simulink model "Reflex_Ursino"  (Simulink 6.4)
settings: Solver=ode45  StartTime=0.0  StopTime=10.0  RelTol=1e-3
values from neighbouring files (symbols this model uses):
  fapIC = 4.4492    [Reflex_Ursino_IC.m]    (also in Respiratory_IC.m)
  fcs_max = 47.78    [Cardiovascular_IC.m]    (also in Reflex_Ursino_IC.m)
  fcs_min = 2.52    [Cardiovascular_IC.m]    (also in Reflex_Ursino_IC.m)
  k_cs = 11.758    [Cardiovascular_IC.m]    (also in Reflex_Ursino_IC.m)
  Pn = 90    [Cardiovascular_IC.m]    (also in Reflex_Ursino_IC.m)
settings Model: LastModifiedBy=CLM
settings OptimizationCC: BlockReduction=off  BooleanDataType=off
settings DebuggingCC: SolverPrmCheckMsg=none  StrictBusMsg=None
settings HardwareCC: TargetUnknown=on

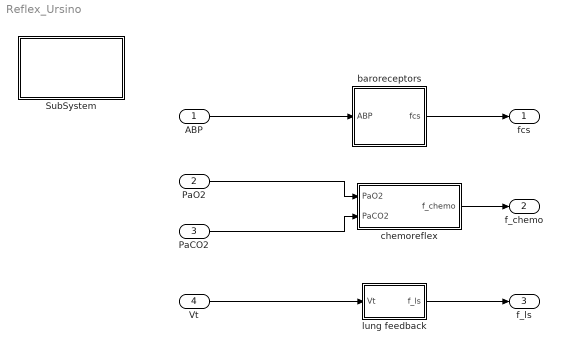
== system Reflex_Ursino ==
  ABP : Inport
  PaO2 : Inport  Port=2
  PaCO2 : Inport  Port=3
  Vt : Inport  Port=4
  SubSystem : Subsystem
      settings: OpenFcn=Reflex_Ursino_IC
      mask Display: disp('"double click here"\n to load \nReflex_Ursino \ninitial values');
  baroreceptors : Subsystem
  chemoreflex : Subsystem
  lung feedback : Subsystem
  fcs : Outport
  f_chemo : Outport  Port=2
  f_ls : Outport  Port=3
  wires:
  baroreceptors/1(fcs) -> fcs/1
  ABP/1 -> baroreceptors/1(ABP)
  chemoreflex/1(f_chemo) -> f_chemo/1
  PaCO2/1 -> chemoreflex/2(PaCO2)
  PaO2/1 -> chemoreflex/1(PaO2)
  Vt/1 -> lung feedback/1(Vt)
  lung feedback/1(f_ls) -> f_ls/1

== system Reflex_Ursino/SubSystem ==

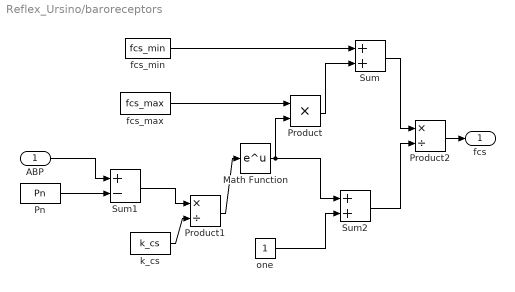
== system Reflex_Ursino/baroreceptors ==
  ABP : Inport
  Math Function : Math  SaturateOnIntegerOverflow=on
  Pn : Constant  Value=Pn  OutDataType=sfix(16)  ConRadixGroup=Use specified scaling  OutScaling=2^0  SampleTime=inf  FramePeriod=inf
  Product : Product  SaturateOnIntegerOverflow=on  RndMeth=Zero  InputSameDT=on
  Product1 : Product  Inputs=*/  SaturateOnIntegerOverflow=on  RndMeth=Zero  InputSameDT=on
  Product2 : Product  Inputs=*/  SaturateOnIntegerOverflow=on  RndMeth=Zero  InputSameDT=on
  Sum : Sum  SaturateOnIntegerOverflow=on  InputSameDT=on
  Sum1 : Sum  Inputs=+-  SaturateOnIntegerOverflow=on  InputSameDT=on
  Sum2 : Sum  SaturateOnIntegerOverflow=on  InputSameDT=on
  fcs_max : Constant  Value=fcs_max  OutDataType=sfix(16)  ConRadixGroup=Use specified scaling  OutScaling=2^0  SampleTime=inf  FramePeriod=inf
  fcs_min : Constant  Value=fcs_min  OutDataType=sfix(16)  ConRadixGroup=Use specified scaling  OutScaling=2^0  SampleTime=inf  FramePeriod=inf
  k_cs : Constant  Value=k_cs  OutDataType=sfix(16)  ConRadixGroup=Use specified scaling  OutScaling=2^0  SampleTime=inf  FramePeriod=inf
  one : Constant  Value=1  OutDataType=sfix(16)  ConRadixGroup=Use specified scaling  OutScaling=2^0  SampleTime=inf  FramePeriod=inf
  fcs : Outport
  wires:
  Sum1/1 -> Product1/1
  Product2/1 -> fcs/1
  Product/1 -> Sum/2
  Sum2/1 -> Product2/2
  Sum/1 -> Product2/1
  one/1 -> Sum2/2
  Math Function/1 -> Sum2/1, Product/2
  Product1/1 -> Math Function/1
  k_cs/1 -> Product1/2
  fcs_max/1 -> Product/1
  fcs_min/1 -> Sum/1
  Pn/1 -> Sum1/2
  ABP/1 -> Sum1/1

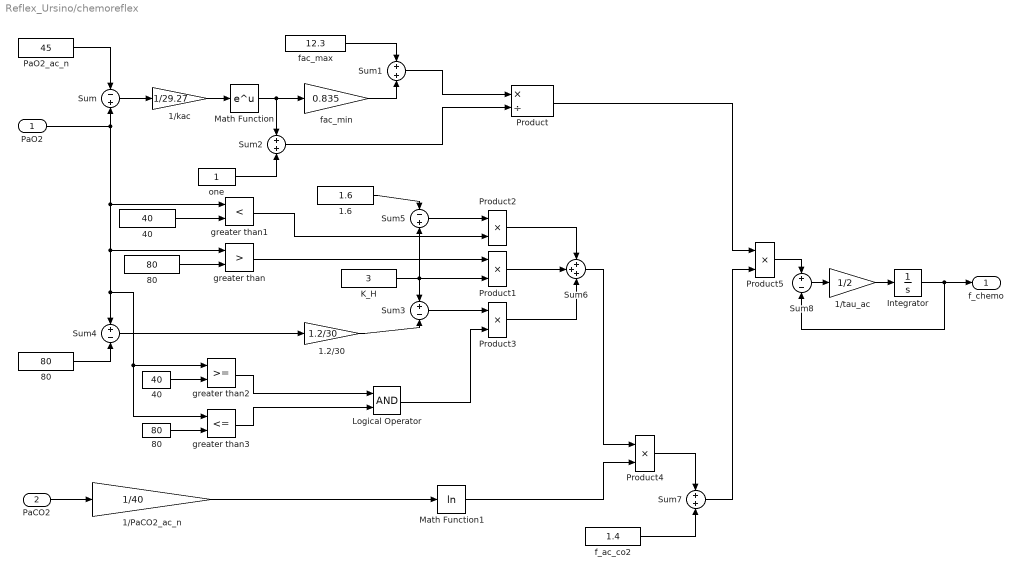
== system Reflex_Ursino/chemoreflex ==
  PaO2 : Inport
  PaCO2 : Inport  Port=2
  "  40  " : Constant  Value=40  OutDataType=sfix(16)  ConRadixGroup=Use specified scaling  OutScaling=2^0  SampleTime=inf  FramePeriod=inf
  "  80  " : Constant  Value=80  OutDataType=sfix(16)  ConRadixGroup=Use specified scaling  OutScaling=2^0  SampleTime=inf  FramePeriod=inf
  " 80 " : Constant  Value=80  OutDataType=sfix(16)  ConRadixGroup=Use specified scaling  OutScaling=2^0  SampleTime=inf  FramePeriod=inf
  1.2/30 : Gain  Gain=1.2/30  SaturateOnIntegerOverflow=on
  1.6 : Constant  Value=1.6  OutDataType=sfix(16)  ConRadixGroup=Use specified scaling  OutScaling=2^0  SampleTime=inf  FramePeriod=inf
  1/PaCO2_ac_n : Gain  Gain=1/40  SaturateOnIntegerOverflow=on
  1/kac : Gain  Gain=1/29.27  SaturateOnIntegerOverflow=on
  1/tau_ac : Gain  Gain=1/2  SaturateOnIntegerOverflow=on
  40 : Constant  Value=40  OutDataType=sfix(16)  ConRadixGroup=Use specified scaling  OutScaling=2^0  SampleTime=inf  FramePeriod=inf
  80 : Constant  Value=80  OutDataType=sfix(16)  ConRadixGroup=Use specified scaling  OutScaling=2^0  SampleTime=inf  FramePeriod=inf
  Integrator : Integrator  InitialCondition=8.0807
  K_H : Constant  Value=3  OutDataType=sfix(16)  ConRadixGroup=Use specified scaling  OutScaling=2^0  SampleTime=inf  FramePeriod=inf
  Logical Operator : Logic
  Math Function : Math  SaturateOnIntegerOverflow=on
  Math Function1 : Math  Operator=log  SaturateOnIntegerOverflow=on
  PaO2_ac_n : Constant  Value=45  OutDataType=sfix(16)  ConRadixGroup=Use specified scaling  OutScaling=2^0  SampleTime=inf  FramePeriod=inf
  Product : Product  Inputs=*/  SaturateOnIntegerOverflow=on  RndMeth=Zero  InputSameDT=on
  Product{1..5} (5 alike) : Product  Inputs=**  SaturateOnIntegerOverflow=on  RndMeth=Zero  InputSameDT=on
  Sum : Sum  Inputs=-+  SaturateOnIntegerOverflow=on  InputSameDT=on
  Sum1 : Sum  SaturateOnIntegerOverflow=on  InputSameDT=on
  Sum2 : Sum  SaturateOnIntegerOverflow=on  InputSameDT=on
  Sum3 : Sum  Inputs=+-  SaturateOnIntegerOverflow=on  InputSameDT=on
  Sum4 : Sum  Inputs=+-  SaturateOnIntegerOverflow=on  InputSameDT=on
  Sum5 : Sum  Inputs=-+  SaturateOnIntegerOverflow=on  InputSameDT=on
  Sum6 : Sum  Inputs=+++  SaturateOnIntegerOverflow=on  InputSameDT=on
  Sum7 : Sum  SaturateOnIntegerOverflow=on  InputSameDT=on
  Sum8 : Sum  Inputs=+-  SaturateOnIntegerOverflow=on  InputSameDT=on
  f_ac_co2 : Constant  Value=1.4  OutDataType=sfix(16)  ConRadixGroup=Use specified scaling  OutScaling=2^0  SampleTime=inf  FramePeriod=inf
  fac_max : Constant  Value=12.3  OutDataType=sfix(16)  ConRadixGroup=Use specified scaling  OutScaling=2^0  SampleTime=inf  FramePeriod=inf
  fac_min : Gain  Gain=0.835  SaturateOnIntegerOverflow=on
  greater than : RelationalOperator  Operator=>  InputSameDT=on
  greater than1 : RelationalOperator  Operator=<  InputSameDT=on
  greater than2 : RelationalOperator  InputSameDT=on
  greater than3 : RelationalOperator  Operator=<=  InputSameDT=on
  one : Constant  Value=1  OutDataType=sfix(16)  ConRadixGroup=Use specified scaling  OutScaling=2^0  SampleTime=inf  FramePeriod=inf
  f_chemo : Outport
  wires:
  Sum/1 -> 1/kac/1
  1/kac/1 -> Math Function/1
  Math Function/1 -> fac_min/1, Sum2/1
  fac_max/1 -> Sum1/1
  fac_min/1 -> Sum1/2
  one/1 -> Sum2/2
  Sum1/1 -> Product/1
  Sum2/1 -> Product/2
  PaO2_ac_n/1 -> Sum/1
  PaO2/1 -> Sum/2, greater than/1, Sum4/1, greater than2/1, greater than3/1, greater than1/1
  80/1 -> Sum4/2
  Sum4/1 -> 1.2/30/1
  1.2/30/1 -> Sum3/2
  Sum3/1 -> Product3/1
  1.6/1 -> Sum5/1
  Sum5/1 -> Product2/1
  K_H/1 -> Sum3/1, Sum5/2, Product1/2
  "  80  "/1 -> greater than/2
  greater than/1 -> Product1/1
  40/1 -> greater than1/2
  greater than1/1 -> Product2/2
  greater than2/1 -> Logical Operator/1
  greater than3/1 -> Logical Operator/2
  Logical Operator/1 -> Product3/2
  " 80 "/1 -> greater than3/2
  "  40  "/1 -> greater than2/2
  Product2/1 -> Sum6/1
  Product1/1 -> Sum6/2
  Product3/1 -> Sum6/3
  PaCO2/1 -> 1/PaCO2_ac_n/1
  1/PaCO2_ac_n/1 -> Math Function1/1
  Sum6/1 -> Product4/1
  Math Function1/1 -> Product4/2
  Product4/1 -> Sum7/1
  f_ac_co2/1 -> Sum7/2
  Product/1 -> Product5/1
  Sum7/1 -> Product5/2
  Product5/1 -> Sum8/1
  Integrator/1 -> f_chemo/1, Sum8/2
  1/tau_ac/1 -> Integrator/1
  Sum8/1 -> 1/tau_ac/1

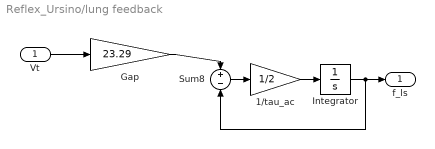
== system Reflex_Ursino/lung feedback ==
  Vt : Inport
  1/tau_ac : Gain  Gain=1/2  SaturateOnIntegerOverflow=on
  Gap : Gain  Gain=23.29  SaturateOnIntegerOverflow=on
  Integrator : Integrator  InitialCondition=fapIC
  Sum8 : Sum  Inputs=+-  SaturateOnIntegerOverflow=on  InputSameDT=on
  f_ls : Outport
  wires:
  Vt/1 -> Gap/1
  Sum8/1 -> 1/tau_ac/1
  1/tau_ac/1 -> Integrator/1
  Integrator/1 -> Sum8/2, f_ls/1
  Gap/1 -> Sum8/1
